simulink model "aprilTagModel"  (R2018a)
settings: Solver=VariableStepAuto  StartTime=0.0  StopTime=10.0  RelTol=1e-3
libraries: visionsources x1
settings Model: Creator=zack  LastModifiedBy=zack
settings OptimizationCC: BlockReduction=off  ConditionallyExecuteInputs=off  DefaultParameterBehavior=Inlined
settings DebuggingCC: AlgebraicLoopMsg=error
settings HardwareCC: ProdBitPerPointer=32  ProdBitPerSizeT=32  ProdBitPerPtrDiffT=32  ProdLargestAtomicFloat=None  ProdIntDivRoundTo=Undefined  ProdEndianess=Unspecified  ProdWordSize=32  ProdHWDeviceType=ASIC/FPGA->ASIC/FPGA  TargetBitPerPointer=64  TargetBitPerSizeT=64  TargetBitPerPtrDiffT=64  TargetLongLongMode=on  TargetIntDivRoundTo=Zero  TargetEndianess=LittleEndian  TargetWordSize=64  TargetHWDeviceType=Custom Processor->MATLAB Host Computer  ProdEqTarget=off

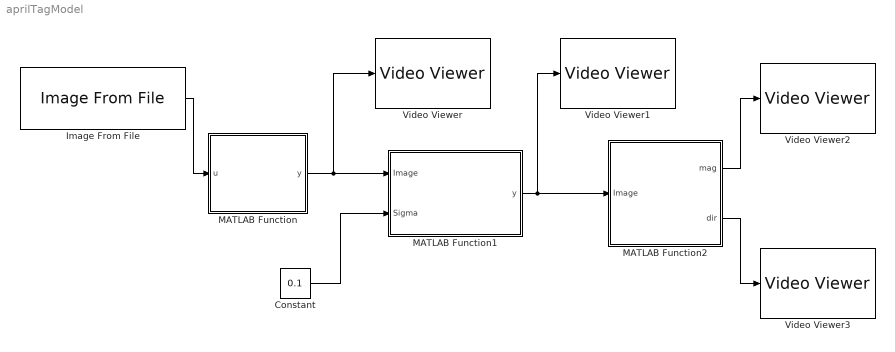
== system aprilTagModel ==
  Constant : Constant  Value=0.1  OutDataTypeStr=fixdt(1,16)
  Image From File : visionsources/Image From File  Tag=vipblks_nd  FileName=C:\Users\zack\Documents\Class_Code\aprilTags\test_tag.png  imagePorts=One multidimensional signal  Ts=inf  ImageDataType=Inherit from input image  Signed=on  WordLength=16  sdImageDataType=uint(8)  FractionLengthMode=User-defined  FractionLength=15  OutPortLabels=R|G|B
      settings: SourceProductName=Computer Vision System Toolbox
  MATLAB Function : MATLAB Function  TreatAsAtomicUnit=on
  MATLAB Function1 : MATLAB Function  TreatAsAtomicUnit=on
  MATLAB Function2 : MATLAB Function  TreatAsAtomicUnit=on
  Video Viewer : VideoViewer  FigPos=[154 520 558 384]
  Video Viewer1 : VideoViewer  FigPos=[738 519 558 384]
  Video Viewer2 : VideoViewer  FigPos=[154 883 560 523]
  Video Viewer3 : VideoViewer  FigPos=[738 796 579 453]
  wires:
  MATLAB Function/1(y) -> Video Viewer/1, MATLAB Function1/1(Image)
  Image From File/1 -> MATLAB Function/1(u)
  Constant/1 -> MATLAB Function1/2(Sigma)
  MATLAB Function1/1(y) -> MATLAB Function2/1(Image), Video Viewer1/1
  MATLAB Function2/1(mag) -> Video Viewer2/1
  MATLAB Function2/2(dir) -> Video Viewer3/1

== matlab function aprilTagModel/MATLAB Function1 ==
  data: Image input; y output; Sigma input
function y = GaussianSmoothing(Image,Sigma)
y = imgaussfilt(Image,0.1);

== matlab function aprilTagModel/MATLAB Function ==
  data: u input; y output
function y = ConvertToGray(u)
y = u(:,:,1)*0.2989 + u(:,:,2)*0.5870 + u(:,:,3)*0.1140;

== matlab function aprilTagModel/MATLAB Function2 ==
  data: Image input; mag output; dir output
function [mag, dir] = LocalGradient(Image)
[height,width,channels] = size(Image);
mag = zeros(height,width); %create an array of zeros to hold magnitude
dir = zeros(height,width); %create an array of zeros to hold direction
G = fspecial('gaussian',3,0.8);
[dx, dy] = gradient(G);
Ix = conv2(Image,dx,'same');
%Ix = NormalizeVals(Ix);
Iy = conv2(Image,dy,'same');
%Iy = NormalizeVals(Iy);
gm = sqrt(Ix.^2 + Iy.^2);
gd = atan2(Iy,Ix);
mag = NormalizeVals(gm);
dir = NormalizeVals(gd);

end

function output = NormalizeVals(input)
output = (input-min(input(:)))./(max(input(:))-min(input(:)));
end
